simulink model "simulink_PD_controller_ubuntu"  (R2024a)
settings: Solver=VariableStepAuto  StartTime=0.0  StopTime=20  RelTol=1e-8
libraries: robotlib x3, simulink x3
settings Model: Creator=ganes  LastModifiedBy=ganesh
settings RTWCC: GPUComputeCapability=3.5

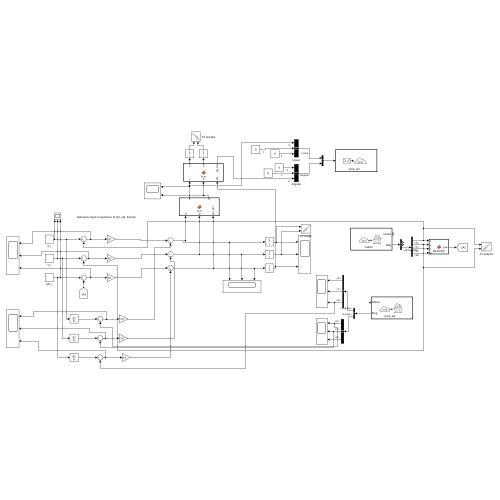
[thumbnail: Simulink's stored preview of the top-level diagram]
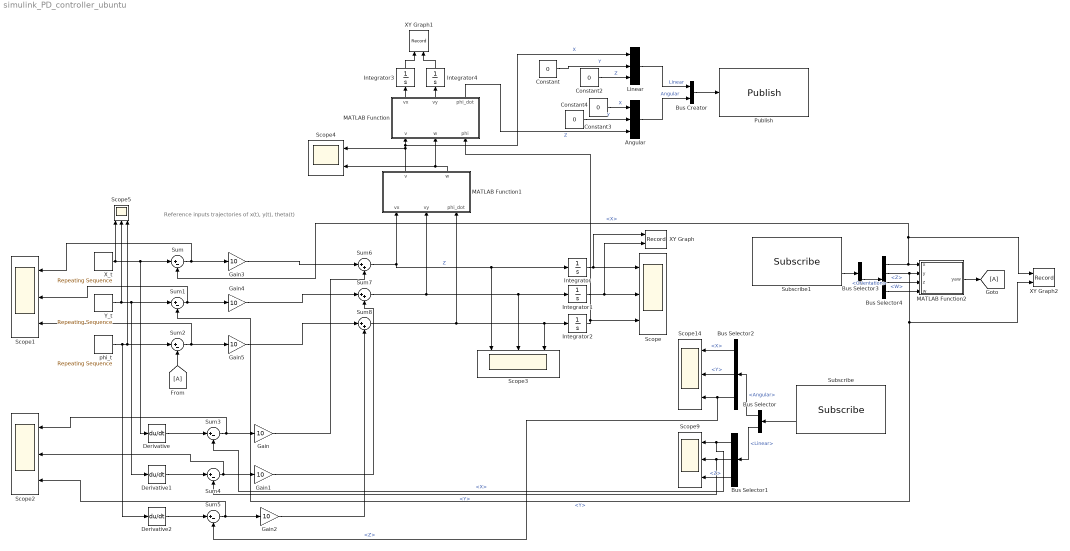
== system simulink_PD_controller_ubuntu ==
  note: Reference inputs trajectories of x(t), y(t), theta(t)
  "Angular " : BusCreator  Inputs=3  OutDataTypeStr=Bus: SL_Bus_simulink_PD_controller_geometry_msgs_Vector3
  Bus Creator : BusCreator  Inputs=2  OutDataTypeStr=Bus: SL_Bus_simulink_PD_controller_geometry_msgs_Twist  NonVirtualBus=on
  Bus Selector : BusSelector  OutputSignals=Angular,Linear
  Bus Selector1 : BusSelector  OutputSignals=X,Y,Z
  Bus Selector2 : BusSelector  OutputSignals=X,Y,Z
  Bus Selector3 : BusSelector  OutputSignals=Pose.Pose.Position,ChildFrameId,Pose.Pose.Orientation
  Bus Selector4 : BusSelector  OutputSignals=X,Y,Z,W
  Constant{,2..4} (4 alike) : Constant  Value=0
  Derivative : Derivative
  Derivative1 : Derivative
  Derivative2 : Derivative
  From : From
  Gain{,1..5} (6 alike) : Gain  Gain=10
  Goto : Goto
  Integrator{,1..4} (5 alike) : Integrator
  Linear : BusCreator  Inputs=3
  MATLAB Function : MATLAB Function  TreatAsAtomicUnit=on
  MATLAB Function1 : MATLAB Function  TreatAsAtomicUnit=on
  MATLAB Function2 : MATLAB Function  TreatAsAtomicUnit=on
  Publish : robotlib/Publish  topicSource=Select from ROS network  topic=/cmd_vel  messageType=geometry_msgs/Twist  legacyBusStruct=off  messageQueueLength=1
  Scope{,1..3,5,9,14} (7 alike) : Scope  NumInputPorts=3
  Scope4 : Scope  NumInputPorts=2
  Subscribe : robotlib/Subscribe  topicSource=Select from ROS network  topic=/cmd_vel  messageType=geometry_msgs/Twist  SampleTime=-1  legacyBusStruct=off  messageQueueLength=1
  Subscribe1 : robotlib/Subscribe  topicSource=Select from ROS network  topic=/odom  messageType=nav_msgs/Odometry  SampleTime=-1  legacyBusStruct=off  messageQueueLength=1
  Sum{,1..5} (6 alike) : Sum  Inputs=|+-
  Sum6 : Sum  Inputs=|++
  Sum7 : Sum  Inputs=|++
  Sum8 : Sum  Inputs=|++
  XY Graph : Record  FileSettingsInternal="{\"entries\":[{\"content\":{\"excelSettings\":{\"content\":{},\"type\":\"Streamout.ExcelSettings\"}},\"type\":\"Streamout.FileSettingStorage\",\"uuid\":\"\"}],\"packageUris\":[\"http:\\/\\/schema.mathworks.com\\/mf0\\/streamout_blocks\\/R2020a\"],\"version\":\"1.0\"}"  Layout=[1 1]  SignalsInternal="{\"entries\":[{\"content\":{\"signals\":[{\"content\":{\"blockPath\":[],\"dimensions\":[1],\"domain\":\"\",\"lineColor\":\"#0072bd\",\"lineWidth\":2,\"port\":1,\"signalID\":1,\"signalName\":\"Integrator\"},\"type\":\"RecordBlkView.Signal\",\"uuid\":\"\"},{\"content\":{\"blockPath\":[],\"dimensions\":[1],\"domain\":\"\",\"lineColor\":\"#d95319\",\"lineWidth\":2,\"port\":2,\"signalID\":2,\"signalName\":\"Integrator1\"},\"type\":\"RecordBlkView.Signal\",\"uuid\":\"\"}]},\"type\":\"RecordBlkView.InputSignals\",\"uuid\":\"\"}],\"packageUris\":[\"http:\\/\\/schema.mathworks.com\\/mf0\\/streamout_blocks\\/R2020a\"],\"version\":\"1.0\"}"  VisualizationBindings="{\"xyplotplugin\":{\"info\":[{\"series\":[],\"subplotID\":1}]}}"  CompatibilityTag=XY
  XY Graph1 : Record  FileSettingsInternal="{\"entries\":[{\"content\":{\"excelSettings\":{\"content\":{},\"type\":\"Streamout.ExcelSettings\"}},\"type\":\"Streamout.FileSettingStorage\",\"uuid\":\"\"}],\"packageUris\":[\"http:\\/\\/schema.mathworks.com\\/mf0\\/streamout_blocks\\/R2020a\"],\"version\":\"1.0\"}"  Layout=[1 1]  SignalsInternal="{\"entries\":[{\"content\":{\"signals\":[{\"content\":{\"blockPath\":[],\"dimensions\":[1],\"domain\":\"\",\"lineColor\":\"#fe330a\",\"plots\":[ 1 ],\"port\":1,\"signalID\":1,\"signalName\":\"Integrator3\"},\"type\":\"RecordBlkView.Signal\",\"uuid\":\"\"},{\"content\":{\"blockPath\":[],\"dimensions\":[1],\"domain\":\"\",\"lineColor\":\"#22b573\",\"port\":2,\"signalID\":2,\"signalName\":\"Integrator4\"},\"type\":\"RecordBlkView.Signal\",\"uuid\":\"\"}]},\"type\":\"RecordBlkView.InputSignals\",\"uuid\":\"\"}],\"packageUris\":[\"http:\\/\\/schema.mathworks.com\\/mf0\\/streamout_blocks\\/R2020a\"],\"version\":\"1.0\"}"  VisualizationBindings="{\"xyplotplugin\":{\"info\":[{\"series\":[{\"bindingParametersList\":[{\"parameter\":\"Y-Axis\",\"signalID\":1,\"signalName\":\"Integrator3\"}],\"seriesID\":0}],\"subplotID\":1}]}}"  CompatibilityTag=XY
  XY Graph2 : Record  FileSettingsInternal="{\"entries\":[{\"content\":{\"excelSettings\":{\"content\":{},\"type\":\"Streamout.ExcelSettings\"}},\"type\":\"Streamout.FileSettingStorage\",\"uuid\":\"\"}],\"packageUris\":[\"http:\\/\\/schema.mathworks.com\\/mf0\\/streamout_blocks\\/R2020a\"],\"version\":\"1.0\"}"  Layout=[1 1]  SignalsInternal="{\"entries\":[{\"content\":{\"signals\":[{\"content\":{\"blockPath\":[],\"dimensions\":[1],\"domain\":\"\",\"lineColor\":\"#fe330a\",\"plots\":[ 1 ],\"port\":1,\"signalID\":1,\"signalName\":\"<X>\"},\"type\":\"RecordBlkView.Signal\",\"uuid\":\"\"},{\"content\":{\"blockPath\":[],\"dimensions\":[1],\"domain\":\"\",\"lineColor\":\"#22b573\",\"port\":2,\"signalID\":2,\"signalName\":\"<Y>\"},\"type\":\"RecordBlkView.Signal\",\"uuid\":\"\"}]},\"type\":\"RecordBlkView.InputSignals\",\"uuid\":\"\"}],\"packageUris\":[\"http:\\/\\/schema.mathworks.com\\/mf0\\/streamout_blocks\\/R2020a\"],\"version\":\"1.0\"}"  VisualizationBindings="{\"xyplotplugin\":{\"info\":[{\"series\":[{\"bindingParametersList\":[{\"parameter\":\"Y-Axis\",\"signalID\":1,\"signalName\":\"<X>\"}],\"seriesID\":0}],\"subplotID\":1}]}}"  CompatibilityTag=XY
  X_t : simulink/Sources/Repeating Sequence  rep_seq_t=t_vec  rep_seq_y=x_t
  Y_t : simulink/Sources/Repeating Sequence  rep_seq_t=t_vec  rep_seq_y=y_t
  phi_t : simulink/Sources/Repeating Sequence  rep_seq_t=t_vec  rep_seq_y=w
  wires:
  Sum7/1 -> Integrator1/1, Scope3/2, MATLAB Function1/2(vy)
  Integrator2/1 -> Scope/3, MATLAB Function/3(phi)
  Integrator/1 -> Scope/1, XY Graph/1
  Integrator1/1 -> XY Graph/2, Scope/2
  phi_t/1 -> Scope5/3, Sum2/1, Derivative2/1
  Y_t/1 -> Derivative1/1, Sum1/1, Scope5/2
  Derivative/1 -> Sum3/1
  Derivative1/1 -> Sum4/1
  Derivative2/1 -> Sum5/1
  Sum/1 -> Scope1/1, Gain3/1
  Sum1/1 -> Scope1/2, Gain4/1
  Sum3/1 -> Scope2/1, Gain/1
  Sum4/1 -> Scope2/2, Gain1/1
  Sum5/1 -> Scope2/3, Gain2/1
  Gain2/1 -> Sum8/2
  Gain1/1 -> Sum7/2
  Gain/1 -> Sum6/2
  Gain4/1 -> Sum7/1
  Gain5/1 -> Sum8/1
  Gain3/1 -> Sum6/1
  Sum2/1 -> Scope1/3, Gain5/1
  MATLAB Function1/2(w) -> MATLAB Function/2(w), Scope4/2
  X_t/1 -> Derivative/1, Sum/1, Scope5/1
  MATLAB Function/1(vx) -> Integrator3/1
  MATLAB Function/2(vy) -> Integrator4/1
  Integrator3/1 -> XY Graph1/1
  Integrator4/1 -> XY Graph1/2
  MATLAB Function1/1(v) -> Linear/1, MATLAB Function/1(v), Scope4/1  "X"
  Bus Creator/1 -> Publish/1
  Sum6/1 -> Integrator/1, Scope3/1, MATLAB Function1/1(vx)  "Z"
  Constant3/1 -> "Angular "/1  "X"
  Constant4/1 -> "Angular "/2  "Y"
  "Angular "/1 -> Bus Creator/2  "Angular"
  Linear/1 -> Bus Creator/1  "Linear"
  Constant2/1 -> Linear/3  "Z"
  Constant/1 -> Linear/2  "Y"
  Sum8/1 -> MATLAB Function1/3(phi_dot), Integrator2/1, Scope3/3
  MATLAB Function/3(phi_dot) -> "Angular "/3  "Z"
  Subscribe1/2 -> Bus Selector3/1
  Bus Selector2/3 -> Sum5/2, Scope14/3  "<Z>"
  Bus Selector2/1 -> Scope14/1  "<X>"
  Bus Selector4/4 -> MATLAB Function2/4(w)  "<W>"
  Bus Selector4/1 -> MATLAB Function2/1(x), XY Graph2/1, Sum/2  "<X>"
  Bus Selector1/2 -> Scope9/2, Sum4/2  "<Y>"
  Bus Selector1/3 -> Scope9/3  "<Z>"
  Bus Selector/2 -> Bus Selector1/1  "<Linear>"
  Bus Selector1/1 -> Sum3/2, Scope9/1  "<X>"
  Bus Selector/1 -> Bus Selector2/1  "<Angular>"
  Bus Selector2/2 -> Scope14/2  "<Y>"
  Subscribe/2 -> Bus Selector/1
  MATLAB Function2/1(yaw) -> Goto/1
  Bus Selector3/3 -> Bus Selector4/1  "<Orientation>"
  Bus Selector4/3 -> MATLAB Function2/3(z)  "<Z>"
  Bus Selector4/2 -> XY Graph2/2, Sum1/2, MATLAB Function2/2(y)  "<Y>"
  From/1 -> Sum2/2

== matlab function simulink_PD_controller_ubuntu/MATLAB Function1 ==
  data: vx input; v output; vy input; phi_dot input; w output
function [v, w] = fcn(vx, vy, phi_dot)
    v=sqrt(vx^2+vy^2);
    w=phi_dot;
end

== matlab function simulink_PD_controller_ubuntu/MATLAB Function ==
  data: v input; vx output; w input; phi input; vy output; phi_dot output
function [vx, vy, phi_dot] = fcn(v, w, phi)
    vx=v*cos(phi);
    vy=v*sin(phi);
    phi_dot=w;
end

== matlab function simulink_PD_controller_ubuntu/MATLAB Function2 ==
  data: x input; yaw output; y input; z input; w input
function yaw=quat2eul(x,y,z,w)
eul=quat2eul([w,x,y,z]);
yaw=eul(1);
end
